simulink model "Vehicle_model"  (R2018a)
settings: Solver=FixedStepAuto  StartTime=0.0  StopTime=40  FixedStep=1e-3  RelTol=1e-2
model workspace (MAT data in the model file):
  Af = 4
  Cd = 0.3
  DrCycles.C505 = [0 1 2 3 4 5 6 7 8 9 10 11 ... (1012 elements, 506x2)]
  DrCycles.FTP = [0 1 2 3 4 5 6 7 8 9 10 11 ... (4956 elements, 2478x2)]
  DrCycles.UDDS = [0 1 2 3 4 5 6 7 8 9 10 11 ... (2746 elements, 1373x2)]
  DrCycles.HWFET = [0 1 2 3 4 5 6 7 8 9 10 11 ... (1532 elements, 766x2)]
  DrCycles.US06 = [0 1 2 3 4 5 6 7 8 9 10 11 ... (1194 elements, 597x2)]
  DrCycles.US06City = [0 1 2 3 4 5 6 7 8 9 10 11 ... (466 elements, 233x2)]
  DrCycles.US06Hwy = [0 1 2 3 4 5 6 7 8 9 10 11 ... (742 elements, 371x2)]
  I = 1
  Kbr = 5000
  P = 20
  Sig = Simulink.Signal
  Sig.DataType = 'auto'
  Sig.Dimensions = -1
  Sig.DimensionsMode = 'auto'
  Sig.Complexity = 'auto'
  Sig.SampleTime = -1
  Sig.SamplingMode = 'auto'
  TimeHWFET = 765
  TimeUDDS = 1372
  TimeUS06 = 596
  axle_b = 10
  axle_k = 5000
  bevAxle_wc = 400
  bevNp = 2
  bevNs = 30
  diffRatio = 3.4
  diffRatio1 = 3.4
  motorMaxTorqueNm = [500 500 500 500 500 500 416.666666667 357.142857143 312.5 277.777777778 250 227.272727273 208.333333333 192.307692308 178.571428571 166.666666667]
  motorMaxTorqueNm2 = [220 220 220 220 220 220 198 176 165 154 143 132 121 110 88 66]
  motorSpeedRadPs = [0 40 80 120 160 200 240 280 320 360 400 440 480 520 560 600]
  motorSpeedRadPs2 = [0 84 168 251 335 419 503 586 670 754 838 922 1005 1089 1173 1361]
  vehicleMass = 1500
  wheelRadius = 0.35
undefined symbols (not defined in the file or in its folder): parms, ref, th, vw
libraries: simulink x2, autolibdatasheetbattery x1, autolibmappedmotor x1, autolibsharedcoupling x1, autolibshareddiff x1, autolibshared x1, Wheels_Driver_VehDyn_Lib x1
settings Model: PauseTimes=2  Creator=ogden.michael  LastModifiedBy=yassi
settings SolverCC: ZeroCrossAlgorithm=Adaptive
settings DebuggingCC: AlgebraicLoopMsg=none  IgnoredZcDiagnostic=none
settings CodeAppCC: StateflowObjectComments=on
settings SimscapeCC: SimscapeNormalizeSystem=off

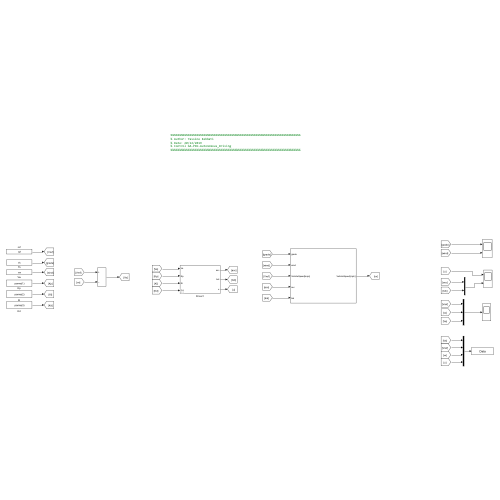
[thumbnail: Simulink's stored preview of the top-level diagram]
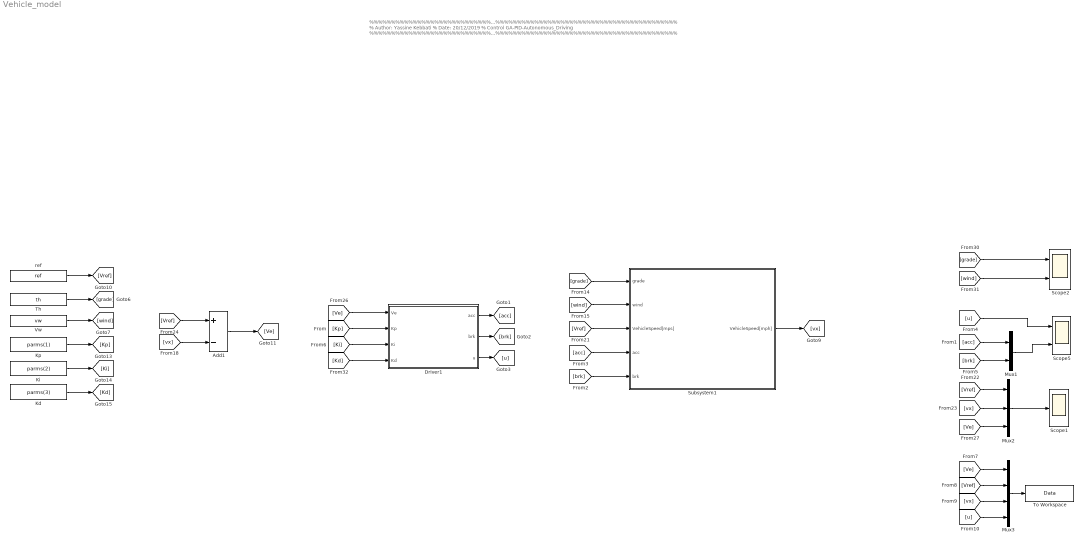
== system Vehicle_model ==
  note: %%%%%%%%%%%%%%%%%%%%%%%%%%%%%%%%%%%%%%%%%%%%%%%%%%%%%%%%%%%%%%%%%%%%%%%%%%%
      | % Author: Yassine Kebbati
      | % Date: 20/12/2019
      | % Control GA-PID-Autonomous_Driving
      | %%%%%%%%%%%%%%%%%%%%%%%%%%%%%%%%%%%%%%%%%%%%%%%%%%%%%%%%%%%%%%%%%%%%%%%%%%%
  Add1 : Sum  Inputs=+-
  Driver1 : Subsystem  AncestorBlock=Wheels_Driver_VehDyn_Lib/Driver
  Kd : Constant  Value=parms(3)
  Ki : Constant  Value=parms(2)
  Kp : Constant  Value=parms(1)
  Mux1 : Mux  Inputs=2
  Mux2 : Mux  Inputs=3
  Mux3 : Mux
  Scope1 : Scope
  Scope2 : Scope  NumInputPorts=2
  Scope5 : Scope  NumInputPorts=2
  Subsystem1 : Subsystem
  Th : Constant  Value=th
  To Workspace : ToWorkspace  VariableName=Data  SaveFormat=Timeseries  SampleTime=-1
  Vw : Constant  Value=vw
  ref : Constant  Value=ref
  wires:
  [Kp] -> Driver1/2(Kp)
  [Ki] -> Driver1/3(Ki)
  [Kd] -> Driver1/4(Kd)
  Mux1/1 -> Scope5/2
  Mux2/1 -> Scope1/1
  [vx] -> Add1/2
  Th/1 -> [grade]
  Driver1/1(acc) -> [acc]
  Driver1/2(brk) -> [brk]
  [acc] -> Subsystem1/4(acc)
  [acc] -> Mux1/1
  [brk] -> Subsystem1/5(brk)
  [brk] -> Mux1/2
  Driver1/3(u) -> [u]
  [grade] -> Subsystem1/1(grade)
  [wind] -> Subsystem1/2(wind)
  Subsystem1/1(VehicleSpeed[mph]) -> [vx]
  [Vref] -> Subsystem1/3(VehicleSpeed[mps])
  [Vref] -> Mux2/1
  [vx] -> Mux2/2
  [Vref] -> Add1/1
  Add1/1 -> [Ve]
  [Ve] -> Driver1/1(Ve)
  [grade] -> Scope2/1
  [wind] -> Scope2/2
  ref/1 -> [Vref]
  Vw/1 -> [wind]
  Kp/1 -> [Kp]
  Ki/1 -> [Ki]
  Kd/1 -> [Kd]
  [u] -> Scope5/1
  [Ve] -> Mux2/3
  Mux3/1 -> To Workspace/1
  [Ve] -> Mux3/1
  [Vref] -> Mux3/2
  [vx] -> Mux3/3
  [u] -> Mux3/4

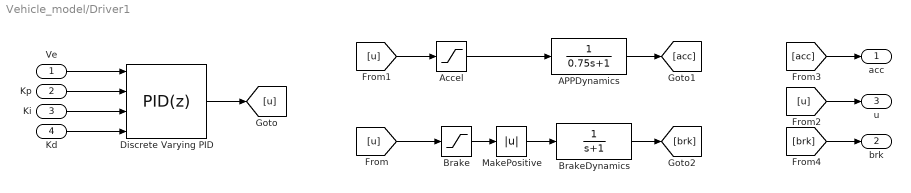
== system Vehicle_model/Driver1 ==
  Ve : Inport
  Kp : Inport  Port=2
  Ki : Inport  Port=3
  Kd : Inport  Port=4
  APPDynamics : TransferFcn  Denominator=[0.75 1]
  Accel : Saturate  UpperLimit=100  LowerLimit=0
  Brake : Saturate  UpperLimit=0  LowerLimit=-100
  BrakeDynamics : TransferFcn  Denominator=[1 1]
  Discrete Varying PID : simulink/Continuous/PID Controller  Controller=PID  Form=Parallel  TimeDomain=Discrete-time  SampleTime=-1  IntegratorMethod=Forward Euler  ControllerParametersSource=external  P=1  I=1  D=0  N=100  UseFilter=off  TunerSelectOption=Transfer Function Based (PID Tuner App)  InitialConditionSource=internal  InitialConditionForIntegrator=0  InitialConditionForFilter=0  DifferentiatorICPrevScaledInput=0  ExternalReset=none  TrackingMode=off  Kt=1  LimitOutput=off  UpperSaturationLimit=100  LowerSaturationLimit=-100  LinearizeAsGain=on  AntiWindupMode=none  Kb=1  POutMin=[]  POutMax=[]  IOutMin=[]  IOutMax=[]  DOutMin=[]  DOutMax=[]  NOutMin=[]  NOutMax=[]  SumOutMin=[]  SumOutMax=[]  SaturationOutMin=[]  SaturationOutMax=[]  PParamMin=[]  PParamMax=[]  IParamMin=[]  IParamMax=[]  DParamMin=[]  DParamMax=[]  NParamMin=[]  NParamMax=[]  KbParamMin=[]  KbParamMax=[]  KtParamMin=[]  KtParamMax=[]  KbOutMin=[]  KbOutMax=[]  KtOutMin=[]  KtOutMax=[]  IntegratorOutMin=[]  IntegratorOutMax=[]  FilterOutMin=[]  FilterOutMax=[]  SumI1OutMin=[]  SumI1OutMax=[]  SumI2OutMin=[]  SumI2OutMax=[]  SumI3OutMin=[]  SumI3OutMax=[]  SumDOutMin=[]  SumDOutMax=[]  DifferentiatorOutMin=[]  DifferentiatorOutMax=[]  FilterDiffOutCoefMin=[]  FilterDiffOutCoefMax=[]  ReciprocalOutMin=[]  ReciprocalOutMax=[]  SumDenOutMin=[]  SumDenOutMax=[]  SumNumOutMin=[]  SumNumOutMax=[]  DivideOutMin=[]  DivideOutMax=[]  IntegratorContinuousStateAttributes=''  IntegratorStateMustResolveToSignalObject=off  IntegratorRTWStateStorageClass=Auto  FilterContinuousStateAttributes=''  FilterStateMustResolveToSignalObject=off  FilterRTWStateStorageClass=Auto
  MakePositive : Abs
  acc : Outport  VectorParamsAs1DForOutWhenUnconnected=off
  brk : Outport  Port=2  VectorParamsAs1DForOutWhenUnconnected=off
  u : Outport  Port=3  VectorParamsAs1DForOutWhenUnconnected=off
  wires:
  MakePositive/1 -> BrakeDynamics/1
  Ve/1 -> Discrete Varying PID/1
  Accel/1 -> APPDynamics/1
  Kp/1 -> Discrete Varying PID/2
  Kd/1 -> Discrete Varying PID/4
  Ki/1 -> Discrete Varying PID/3
  Brake/1 -> MakePositive/1
  BrakeDynamics/1 -> [brk]
  APPDynamics/1 -> [acc]
  Discrete Varying PID/1 -> [u]
  [u] -> Brake/1
  [u] -> Accel/1
  [u] -> u/1
  [acc] -> acc/1
  [brk] -> brk/1

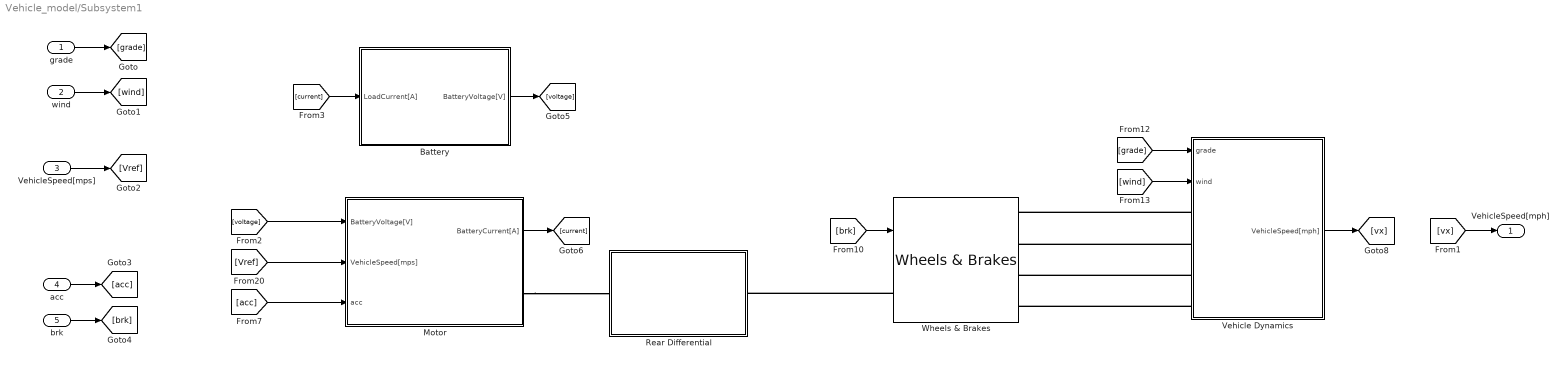
== system Vehicle_model/Subsystem1 ==
  grade : Inport
  wind : Inport  Port=2
  VehicleSpeed[mps] : Inport  Port=3
  acc : Inport  Port=4
  brk : Inport  Port=5
  Battery : Subsystem
  Motor : Subsystem
  Rear Differential : Subsystem
  Vehicle Dynamics : Subsystem  AncestorBlock=Wheels_Driver_VehDyn_Lib/Vehicle Dynamics
  "Wheels & Brakes " : Wheels_Driver_VehDyn_Lib/Wheels & Brakes  SystemSampleTime=-1  Latency=0  AutoFrameSizeCalculation=off
      link override BrakeGain: Gain=Kbr
      link override Longitudinal Wheel - Disk Brake: Re=0.32995  Lrel=0.32995  rollingType=Magic Formula  Iyy=0.798  UNLOADED_RADIUS=0.32995  num_pads=2
      link override Longitudinal Wheel - Disk Brake1: Iyy=0.798  Lrel=0.32995  Re=0.32995  rollingType=Magic Formula  UNLOADED_RADIUS=0.32995
  VehicleSpeed[mph] : Outport
  wires:
  [vx] -> VehicleSpeed[mph]/1
  wind/1 -> [wind]
  [Vref] -> Motor/2(VehicleSpeed[mps])
  [grade] -> Vehicle Dynamics/1(grade)
  [acc] -> Motor/3(acc)
  [current] -> Battery/1(LoadCurrent[A])
  VehicleSpeed[mps]/1 -> [Vref]
  brk/1 -> [brk]
  Motor/1(BatteryCurrent[A]) -> [current]
  [voltage] -> Motor/1(BatteryVoltage[V])
  Vehicle Dynamics/1(VehicleSpeed[mph]) -> [vx]
  [brk] -> "Wheels & Brakes "/1
  [wind] -> Vehicle Dynamics/2(wind)
  grade/1 -> [grade]
  acc/1 -> [acc]
  Battery/1(BatteryVoltage[V]) -> [voltage]
  connections:
  Motor/RConn1 -- Rear Differential/LConn1
  Vehicle Dynamics/LConn4 -- "Wheels & Brakes "/RConn4
  Vehicle Dynamics/LConn3 -- "Wheels & Brakes "/RConn3
  "Wheels & Brakes "/LConn1 -- Rear Differential/RConn1
  Vehicle Dynamics/LConn1 -- "Wheels & Brakes "/RConn1
  Vehicle Dynamics/LConn2 -- "Wheels & Brakes "/RConn2

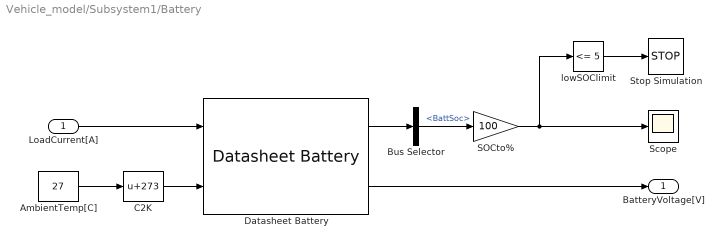
== system Vehicle_model/Subsystem1/Battery ==
  LoadCurrent[A] : Inport
  AmbientTemp[C] : Constant  Value=27
  Bus Selector : BusSelector  OutputSignals=BattSoc
  C2K : Bias  Bias=273
  Datasheet Battery : autolibdatasheetbattery/Datasheet Battery  CapacityCtrl=Parameter  OutputVlt=Unfiltered  BattChargeMax=131.82  Em=[3.167 3.413 3.446 3.488 3.537 3.571 3.593 3.610 3.625 3.642 3.663 3.695 3.755 3.799 3.846 3.895 3.945 3.997 4.051 4.108 4.166]  CapLUTBp=[0 0.05 0.1 0.15 0.2 0.25 0.3 0.35 0.4 0.45 0.5 0.55 0.6 0.65 0.7 0.75 0.8 0.85 0.9 0.95 1]  RInt=[0.008846 0.009319 0.009027 0.00847 0.01032 0.01314;0.006389 0.006554 0.005553 0.005525 0.006043 0.007805;0.004364 0.004101 0.00406 0.003452 0.003846 0.004517;0.002031 0.002563 0.002532 0.00246 0.002716 0.003047;0.001443 0.001825 0.001795 0.001778 0.001924 0.002234;0.0005603 0.0007192 0.0006887 0.0007557 0.0007355 0.001014;0.001028 0.001338 0.001 0.001536 0.001546 0.002789]  BattTempBp=[243.1 253.1 263.1 273.1 283.1 298.1 313.1]  CapSOCBp=[0 0.2 0.4 0.6 0.8 1]  Ns=96  Np=2  BattCapInit=131.82  Tc=1/1000  Vinit=4.221
  SOCto% : Gain  Gain=100
  Scope : Scope
  Stop Simulation : Stop
  lowSOClimit : simulink/Logic and Bit Operations/Compare To Constant  relop=<=  const=5  OutDataTypeStr=boolean
  BatteryVoltage[V] : Outport  VectorParamsAs1DForOutWhenUnconnected=off
  wires:
  Datasheet Battery/1 -> Bus Selector/1
  AmbientTemp[C]/1 -> C2K/1
  Datasheet Battery/2 -> BatteryVoltage[V]/1
  C2K/1 -> Datasheet Battery/2
  SOCto%/1 -> lowSOClimit/1, Scope/1
  Bus Selector/1 -> SOCto%/1  "<BattSoc>"
  LoadCurrent[A]/1 -> Datasheet Battery/1
  lowSOClimit/1 -> Stop Simulation/1

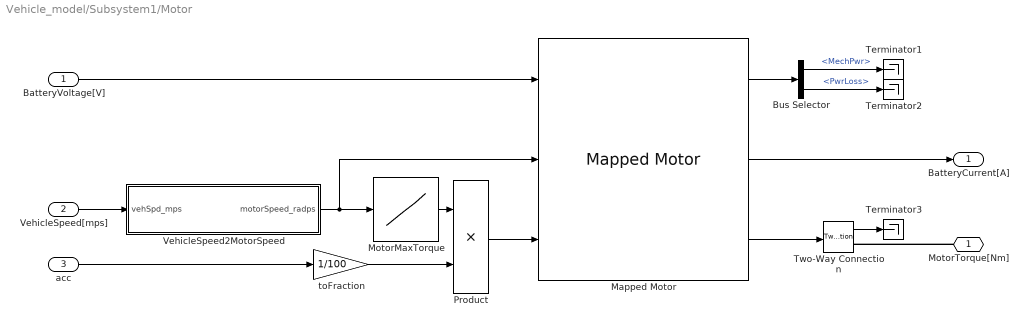
== system Vehicle_model/Subsystem1/Motor ==
  BatteryVoltage[V] : Inport
  VehicleSpeed[mps] : Inport  Port=2
  acc : Inport  Port=3
  Bus Selector : BusSelector  OutputSignals=MechPwr,PwrLoss
  Mapped Motor : autolibmappedmotor/Mapped Motor  port_config=Speed  param_by=Tabulated torque-speed envelope  w_t=motorSpeedRadPs  T_t=motorMaxTorqueNm  torque_max=.1  power_max=30  Tc=0.02  param_loss=Single efficiency measurement  eff=100  w_eff=375  T_eff=0.08  Piron=0  Pbase=0  w_eff_bp=[-8000 -4000 0 4000 8000]  T_eff_bp=[0 0.03 0.06 0.09]  losses_table=[1.49 1.67 2.21 3.10; 0.42 0.69 1.14 2.03; 0.06 0.24 0.78 1.68; 0.42 0.69 1.14 2.03; 1.49 1.67 2.21 3.10]  efficiency_table=[95 95 95 95; 95 95 95 95; 95 95 95 95; 95 95 95 95; 95 95 95 95]  J=5e-6  b=1e-5  omega_o=0  T_t_extended=[166.666666666667 178.571428571429 192.307692307692 208.333333333333 227.272727272727 250 277.777777777778 312.5 357.142857142857 416.666666666667 500 500 500 500 500 500 500 500 500 500 500 416.666666666667 357.142857142857 312.5 277.777777777778 250 227.272727272727 208.333333333333 192.307692307692 178.571428571429 166.666666666667]  w_t_extended=[-600 -560 -520 -480 -440 -400 -360 -320 -280 -240 -200 -160 -120 -80 -40 0 40 80 120 160 200 240 280 320 360 400 440 480 520 560 600]  KLossIron=0  KLossCopper=0  x_w_eff_vec=[-8000 -4000 0 4000 8000]  x_T_eff_vec=[-0.09 -0.06 -0.03 0 0.03 0.06 0.09]  x_losses_mat=[3.1 2.21 1.67 1.49 1.67 2.21 3.1;2.03 1.14 0.69 0.42 0.69 1.14 2.03;1.68 0.78 0.24 0.06 0.24 0.78 1.68;2.03 1.14 0.69 0.42 0.69 1.14 2.03;3.1 2.21 1.67 1.49 1.67 2.21 3.1]  aMode=aMode
  MotorMaxTorque : Lookup_n-D  NumberOfTableDimensions=1  BreakpointsForDimension1=motorSpeedRadPs  Table=motorMaxTorqueNm  ExtrapMethod=Clip  InternalRulePriority=Speed  RndMeth=Simplest  InputSameDT=on
  Product : Product
  Terminator1 : Terminator
  Terminator2 : Terminator
  Terminator3 : Terminator
  Two-Way Connectio n : TwoWayConnection
  VehicleSpeed2MotorSpeed : Subsystem
  toFraction : Gain  Gain=1/100
  MotorTorque[Nm] : PMIOPort  Side=Right
  BatteryCurrent[A] : Outport  VectorParamsAs1DForOutWhenUnconnected=off
  wires:
  BatteryVoltage[V]/1 -> Mapped Motor/1
  Mapped Motor/2 -> BatteryCurrent[A]/1
  VehicleSpeed[mps]/1 -> VehicleSpeed2MotorSpeed/1(vehSpd_mps)
  VehicleSpeed2MotorSpeed/1(motorSpeed_radps) -> MotorMaxTorque/1, Mapped Motor/2
  Mapped Motor/1 -> Bus Selector/1
  Two-Way Connectio n/1 -> Terminator3/1
  Product/1 -> Mapped Motor/3
  MotorMaxTorque/1 -> Product/1
  acc/1 -> toFraction/1
  toFraction/1 -> Product/2
  Bus Selector/2 -> Terminator2/1  "<PwrLoss>"
  Bus Selector/1 -> Terminator1/1  "<MechPwr>"
  Mapped Motor/3 -> Two-Way Connectio n/1
  connections:
  MotorTorque[Nm]/RConn1 -- Two-Way Connectio n/RConn1

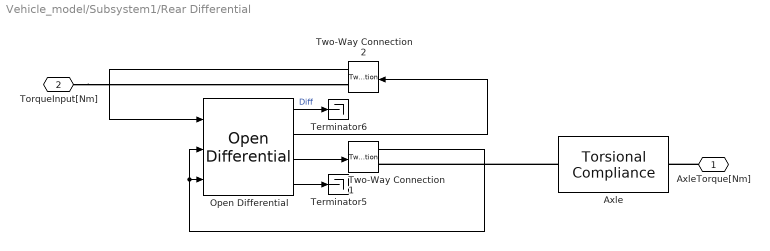
== system Vehicle_model/Subsystem1/Rear Differential ==
  Axle : autolibsharedcoupling/Torsional Compliance  port_config=Two-way connection  k=axle_k  b=axle_b  theta_o=0  domega_o=0  omega_c=bevAxle_wc  blkID=0  aMode=1
  Open Differential : autolibshareddiff/Open Differential  shaftSwitchMask=To the left of center-line  Ndiff=diffRatio  Jd=.025  bd=1e-3  Jw1=.01  bw1=1e-3  Jw2=.01  bw2=1e-3  omegaw1o=0  omegaw2o=0  maxAbsSpd=5e3  aMode=aMode
  Terminator5 : Terminator
  Terminator6 : Terminator
  Two-Way Connection1 : TwoWayConnection
  Two-Way Connection2 : TwoWayConnection
  AxleTorque[Nm] : PMIOPort  Side=Right
  TorqueInput[Nm] : PMIOPort  Port=2  Side=Left
  wires:
  Open Differential/3 -> Two-Way Connection1/1
  Open Differential/4 -> Terminator5/1
  Open Differential/1 -> Terminator6/1  "Diff"
  Open Differential/2 -> Two-Way Connection2/1
  Two-Way Connection1/1 -> Open Differential/2, Open Differential/3
  Two-Way Connection2/1 -> Open Differential/1
  connections:
  Axle/LConn1 -- Two-Way Connection1/RConn1
  TorqueInput[Nm]/RConn1 -- Two-Way Connection2/RConn1
  AxleTorque[Nm]/RConn1 -- Axle/RConn1

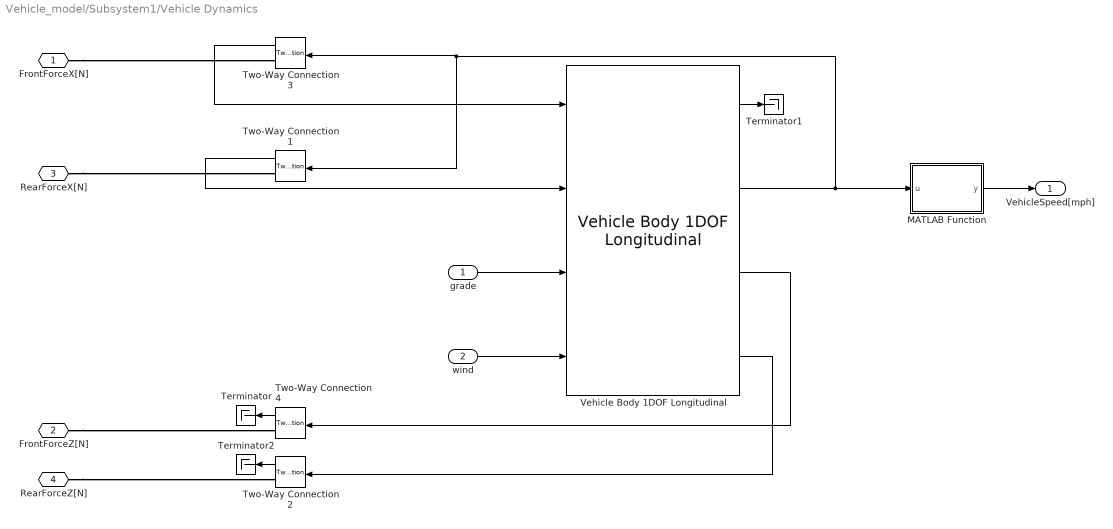
== system Vehicle_model/Subsystem1/Vehicle Dynamics ==
  grade : Inport
  wind : Inport  Port=2
  MATLAB Function : MATLAB Function  TreatAsAtomicUnit=on
  Terminator : Terminator
  Terminator1 : Terminator
  Terminator2 : Terminator
  Two-Way Connection{1..4} (4 alike) : TwoWayConnection
  Vehicle Body 1DOF Longitudinal : autolibshared/Vehicle Body 1DOF Longitudinal  VariantControl=SL  aMode=aMode  NF=2  NR=2  m=1468  a=1.13225  b=1.45575  h=.35  Cd=0.29  Af=2.22  x_o=0  xdot_o=0  Pabs=101325  T=293.15  g=9.81
  FrontForceX[N] : PMIOPort  Side=Left
  FrontForceZ[N] : PMIOPort  Port=2  Side=Left
  RearForceX[N] : PMIOPort  Port=3  Side=Left
  RearForceZ[N] : PMIOPort  Port=4  Side=Left
  VehicleSpeed[mph] : Outport  VectorParamsAs1DForOutWhenUnconnected=off
  wires:
  grade/1 -> Vehicle Body 1DOF Longitudinal/3
  wind/1 -> Vehicle Body 1DOF Longitudinal/4
  Vehicle Body 1DOF Longitudinal/1 -> Terminator1/1
  Vehicle Body 1DOF Longitudinal/3 -> Two-Way Connection4/1
  Vehicle Body 1DOF Longitudinal/4 -> Two-Way Connection2/1
  Two-Way Connection3/1 -> Vehicle Body 1DOF Longitudinal/1
  Two-Way Connection1/1 -> Vehicle Body 1DOF Longitudinal/2
  Two-Way Connection4/1 -> Terminator/1
  Two-Way Connection2/1 -> Terminator2/1
  Vehicle Body 1DOF Longitudinal/2 -> MATLAB Function/1(u), Two-Way Connection1/1, Two-Way Connection3/1
  MATLAB Function/1(y) -> VehicleSpeed[mph]/1
  connections:
  FrontForceX[N]/RConn1 -- Two-Way Connection3/RConn1
  FrontForceZ[N]/RConn1 -- Two-Way Connection4/RConn1
  RearForceX[N]/RConn1 -- Two-Way Connection1/RConn1
  RearForceZ[N]/RConn1 -- Two-Way Connection2/RConn1

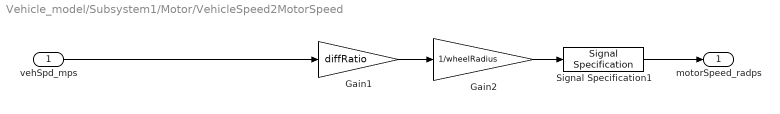
== system Vehicle_model/Subsystem1/Motor/VehicleSpeed2MotorSpeed ==
  vehSpd_mps : Inport
  Gain1 : Gain  Gain=diffRatio
  Gain2 : Gain  Gain=1/wheelRadius
  Signal Specification1 : SignalSpecification  Unit=rad/s
  motorSpeed_radps : Outport  VectorParamsAs1DForOutWhenUnconnected=off
  wires:
  Signal Specification1/1 -> motorSpeed_radps/1
  vehSpd_mps/1 -> Gain1/1
  Gain1/1 -> Gain2/1
  Gain2/1 -> Signal Specification1/1

== matlab function Vehicle_model/Subsystem1/Vehicle Dynamics/MATLAB Function ==
  data: u input; y output
function y = fcn(u)
if u > 10^5;
    u = 10^5;
elseif u < -10^5;
    u=-10^5;
end
y = u;
